simulink model "clase17112020"  (R2020b)
settings: Solver=VariableStepAuto  StartTime=0.0  StopTime=10.0  RelTol=1e-3
libraries: dsparch4 x1, commanapbnd3 x1
settings Model: Creator=fer-1  LastModifiedBy=fer-1

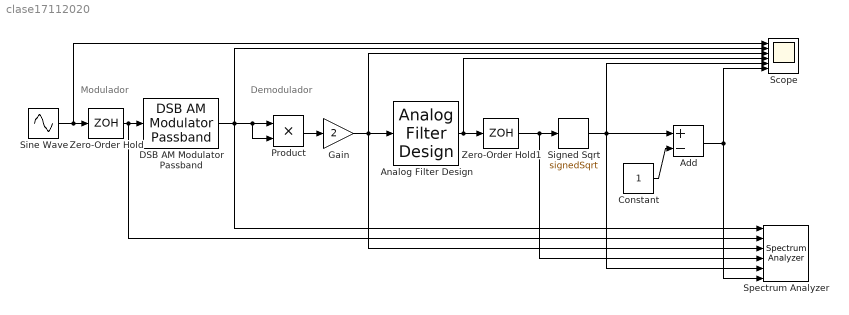
== system clase17112020 ==
  note: Demodulador
  note: Modulador
  Add : Sum  Inputs=+-
  Analog Filter Design : dsparch4/Analog Filter Design  method=Butterworth  filttype=Lowpass  N=8  Wlo=2*pi*10e3  Whi=80  Rp=2  Rs=40
  Constant : Constant
  DSB AM Modulator Passband : commanapbnd3/DSB AM Modulator Passband  Fc=20e3  Ph=0  Offset=1
      settings: SourceProductBaseCode=CM
  Gain : Gain  Gain=2
  Product : Product
  Scope : Scope  NumInputPorts=6
  Signed Sqrt : Sqrt  Operator=signedSqrt  SaturateOnIntegerOverflow=on
  Sine Wave : Sin  Frequency=2*pi*1e3  SampleTime=0
  Spectrum Analyzer : SpectrumAnalyzer  NumInputPorts=6
  Zero-Order Hold : ZeroOrderHold  SampleTime=1/20e2
  Zero-Order Hold1 : ZeroOrderHold  SampleTime=1/20e2
  wires:
  Signed Sqrt/1 -> Spectrum Analyzer/5, Add/1, Scope/5
  Gain/1 -> Analog Filter Design/1, Spectrum Analyzer/3, Scope/3
  Constant/1 -> Add/2
  DSB AM Modulator Passband/1 -> Product/2, Product/1, Spectrum Analyzer/1, Scope/2
  Zero-Order Hold/1 -> Spectrum Analyzer/2, DSB AM Modulator Passband/1
  Zero-Order Hold1/1 -> Signed Sqrt/1, Spectrum Analyzer/4
  Sine Wave/1 -> Scope/1, Zero-Order Hold/1
  Analog Filter Design/1 -> Zero-Order Hold1/1, Scope/4
  Add/1 -> Spectrum Analyzer/6, Scope/6
  Product/1 -> Gain/1
